simulink model "control_core"  (R2022b)
settings: Solver=FixedStepAuto  StartTime=0.0  StopTime=60  FixedStep=.01  RelTol=1e-3
undefined symbols (not defined in the file): airframe, CdProp, Cdx, Cdy, Cdz, Ct, Earth, g, Ixx, Iyy, Izz, Jr, larm, mass, WGS84
libraries: slpidlib x6, aerolibutil x3, vrlib x3, sharedtransform x2, shared6dof x2, simulink_extras x2, simulink x2, aerolibfltsims x1, aerolibtransform2 x1
(part 1 of 2)
settings Model: Creator=aaron  LastModifiedBy=aaron

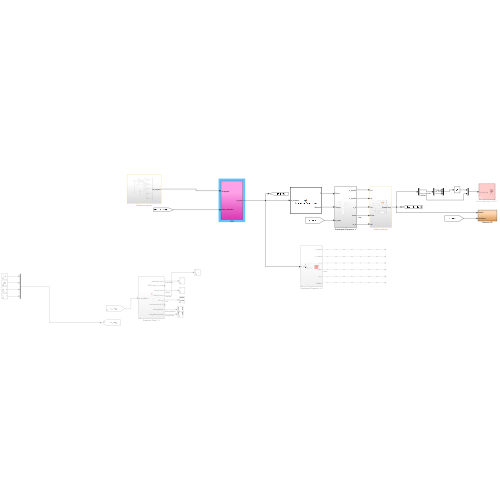
[thumbnail: Simulink's stored preview of the top-level diagram]
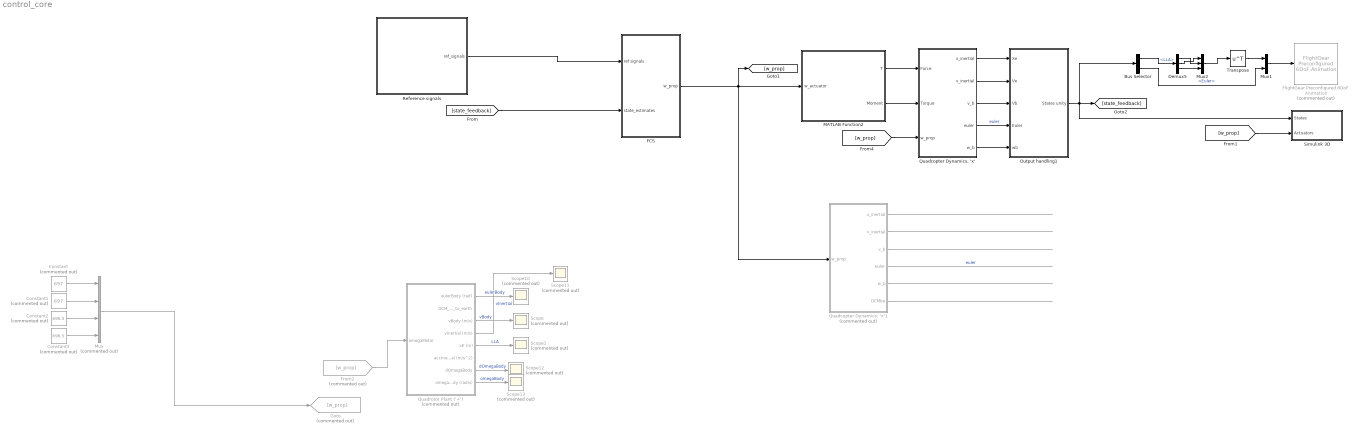
== system control_core ==
  Bus Selector : BusSelector  OutputSignals=LLA,Euler
  Constant : Constant  Commented=on  Value=697
  Constant1 : Constant  Commented=on  Value=697
  Constant2 : Constant  Commented=on  Value=696.5
  Constant3 : Constant  Commented=on  Value=696.5
  Demux5 : Demux  Outputs=3
  FCS : Subsystem
  FlightGear Preconfigured 6DoF Animation : aerolibfltsims/FlightGear Preconfigured 6DoF Animation  Commented=on  xFlightGearVersion=v2019.1  DestinationIpAddress=127.0.0.1  DestinationPort=5502  SampleTime=.0001  packetVersion=24
  From2 : From  Commented=on  GotoTag=w_prop
  Goto : Goto  Commented=on  GotoTag=w_prop
  MATLAB Function2 : MATLAB Function  TreatAsAtomicUnit=on
  Mux : Mux  Commented=on
  Mux1 : Mux  Inputs=2
  Mux2 : Mux  Inputs=3
  Output handling1 : Subsystem
  "Quadcopter Dynamics, 'x'" : Subsystem
  "Quadcopter Dynamics, 'x'1" : Subsystem  Commented=on
  Quadrotor Plant ('+') : Subsystem  Commented=on
  Reference signals : Subsystem
  Scope{,1,10..13} (6 alike) : Scope  Commented=on
  Simulink 3D : Subsystem  VariantControl=VSS_VISUALIZATION==VisualizationMode.Simulink_3D
  Transpose : Math  Operator=transpose
  wires:
  Quadrotor Plant ('+')/3(vBody (m/s)) -> Scope/1  "vBody"
  Quadrotor Plant ('+')/5(xE (m)) -> Scope1/1  "LLA"
  Mux/1 -> Goto/1
  Quadrotor Plant ('+')/1(eulerBody (rad)) -> Scope10/1  "eulerBody"
  Quadrotor Plant ('+')/4(vInertial (m/s)) -> Scope11/1  "vInertial"
  Quadrotor Plant ('+')/7(dOmegaBody) -> Scope12/1  "dOmegaBody"
  Quadrotor Plant ('+')/8(omegaBody (rad/s)) -> Scope13/1  "omegaBody"
  From2/1 -> Quadrotor Plant ('+')/1(omegaMotor)
  Constant/1 -> Mux/1
  Constant1/1 -> Mux/2
  Constant2/1 -> Mux/3
  Constant3/1 -> Mux/4
  "Quadcopter Dynamics, 'x'1"/1(x_inertial) -> ?
  "Quadcopter Dynamics, 'x'1"/2(v_inertial) -> ?
  "Quadcopter Dynamics, 'x'1"/3(v_b) -> ?
  "Quadcopter Dynamics, 'x'1"/4(euler) -> ?  "euler"
  "Quadcopter Dynamics, 'x'1"/5(w_b) -> ?
  "Quadcopter Dynamics, 'x'1"/6(DCMbe) -> ?
  MATLAB Function2/1(T) -> "Quadcopter Dynamics, 'x'"/1(Force)
  MATLAB Function2/2(Moment) -> "Quadcopter Dynamics, 'x'"/2(Torque)
  [w_prop] -> "Quadcopter Dynamics, 'x'"/3(w_prop)
  "Quadcopter Dynamics, 'x'"/1(x_inertial) -> Output handling1/1(Xe)
  "Quadcopter Dynamics, 'x'"/2(v_inertial) -> Output handling1/2(Ve)
  "Quadcopter Dynamics, 'x'"/3(v_b) -> Output handling1/3(Vb)
  "Quadcopter Dynamics, 'x'"/4(euler) -> Output handling1/4(Euler)  "euler"
  "Quadcopter Dynamics, 'x'"/5(w_b) -> Output handling1/5(wb)
  Output handling1/1(States unity) -> [state_feedback], Simulink 3D/1(States), Bus Selector/1
  Mux1/1 -> FlightGear Preconfigured 6DoF Animation/1
  Transpose/1 -> Mux1/1
  Demux5/1 -> Mux2/2
  Demux5/2 -> Mux2/1
  Mux2/1 -> Transpose/1
  Demux5/3 -> Mux2/3
  Bus Selector/1 -> Demux5/1  "<LLA>"
  Bus Selector/2 -> Mux1/2  "<Euler>"
  [w_prop] -> Simulink 3D/2(Actuators)
  FCS/1(w_prop) -> "Quadcopter Dynamics, 'x'1"/1(w_prop), [w_prop], MATLAB Function2/1(w_actuator)
  Reference signals/1(ref_signals) -> FCS/1(ref signals)
  [state_feedback] -> FCS/2(state_estimates)

== system control_core/FCS ==
  ref signals : Inport
  state_estimates : Inport  Port=2
  FCS : Subsystem
  Motor Mixing : Subsystem
  w_prop : Outport
  wires:
  ref signals/1 -> FCS/1(ref signals)
  FCS/2(Torque command) -> Motor Mixing/2(Torque)
  Motor Mixing/1(motor_rpm) -> w_prop/1  "w_prop"
  FCS/1(Force command) -> Motor Mixing/1(Force)
  state_estimates/1 -> FCS/2(state_estimates)

== system control_core/Output handling1 ==
  Xe : Inport
  Ve : Inport  Port=2
  Vb : Inport  Port=3
  Euler : Inport  Port=4
  wb : Inport  Port=5
  Bus Creator : BusCreator  Inputs=7
  Position on Earth : Subsystem  Priority=1  TreatAsAtomicUnit=on
  Rotation Angles to Direction Cosine Matrix : sharedtransform/Rotation Angles to Direction Cosine Matrix  rotationOrder=ZYX  aMode=aMode
  Selector : Selector  InputPortWidth=3  IndexOptions=Index vector (dialog)  Indices=[3 2 1]  OutputSizes=1
  States unity : Outport
  wires:
  Selector/1 -> Rotation Angles to Direction Cosine Matrix/1
  Bus Creator/1 -> States unity/1
  Ve/1 -> Bus Creator/3  "V_inertial"
  Xe/1 -> Position on Earth/1(Xe), Bus Creator/1  "X_inertial_me"
  Vb/1 -> Bus Creator/4  "v_body"
  wb/1 -> Bus Creator/6  "w_body"
  Euler/1 -> Bus Creator/5, Selector/1  "Euler"
  Rotation Angles to Direction Cosine Matrix/1 -> Bus Creator/7  "DCMbe"
  Position on Earth/1(LLA) -> Bus Creator/2  "LLA"

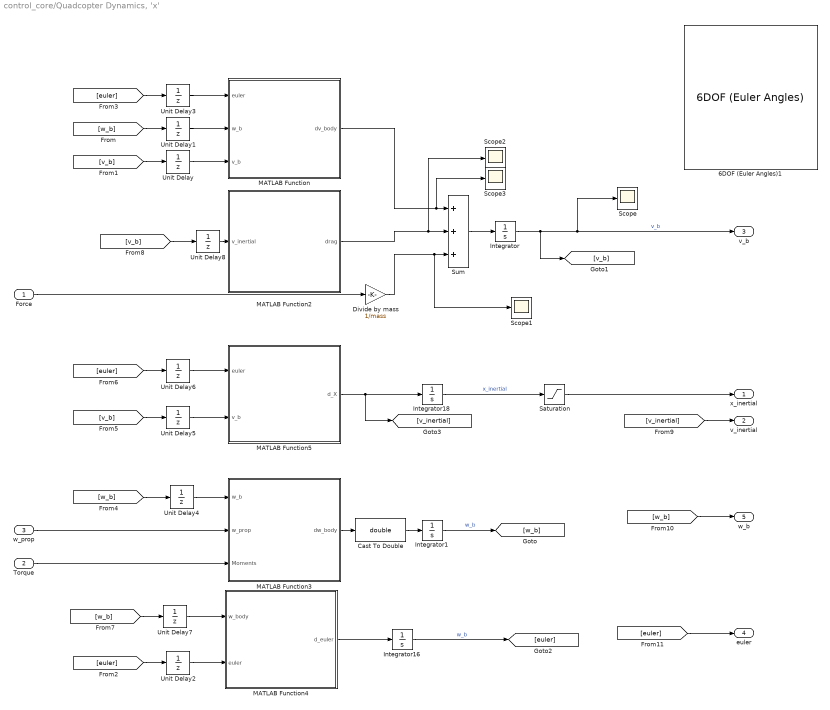
== system control_core/Quadcopter Dynamics, 'x' ==
  Force : Inport
  Torque : Inport  Port=2
  w_prop : Inport  Port=3
  6DOF (Euler Angles)1 : shared6dof/6DOF (Euler Angles)  units=Metric (MKS)  mtype=Fixed  rep=Euler Angles  xme_0=[0 0 0]  Vm_0=[0 0 0]  eul_0=[0 0 0]  pm_0=[0 0 0]  mass_0=1.0  mass_e=0.5  mass_f=2.0  inertia=eye(3)  inertia_e=eye(3)  inertia_f=2*eye(3)  k_quat=1.0  vre_flag=on  abi_flag=off  aMode=0  xme_statename=''  Vm_statename=''  eul_statename=''  quat_statename=''  pm_statename=''  mass_statename=''
  Cast To Double : DataTypeConversion  OutDataTypeStr=double  SaturateOnIntegerOverflow=off  RndMeth=Floor
  Divide by mass : Gain  Gain=1/mass
  Integrator : Integrator
  Integrator1 : Integrator
  Integrator16 : Integrator  InitialCondition=[0 0 0]  WrapState=on
  Integrator18 : Integrator  LimitOutput=on  UpperSaturationLimit=[inf inf 0]  LowerSaturationLimit=[-inf -inf -inf]
  MATLAB Function : MATLAB Function  TreatAsAtomicUnit=on
  MATLAB Function2 : MATLAB Function  TreatAsAtomicUnit=on
  MATLAB Function3 : MATLAB Function  TreatAsAtomicUnit=on
  MATLAB Function4 : MATLAB Function  TreatAsAtomicUnit=on
  MATLAB Function5 : MATLAB Function  TreatAsAtomicUnit=on
  Saturation : Saturate  UpperLimit=[inf inf 0]  LowerLimit=-inf
  Scope{,1..3} (4 alike) : Scope
  Sum : Sum  Inputs=+++
  Unit Delay{,1..8} (9 alike) : UnitDelay  SampleTime=-1  HasFrameUpgradeWarning=on
  x_inertial : Outport
  v_inertial : Outport  Port=2
  v_b : Outport  Port=3
  euler : Outport  Port=4
  w_b : Outport  Port=5
  wires:
  MATLAB Function/1(dv_body) -> Scope3/1, Sum/1
  MATLAB Function2/1(drag) -> Scope2/1, Sum/2
  Unit Delay/1 -> MATLAB Function/3(v_b)
  Force/1 -> Divide by mass/1
  MATLAB Function3/1(dw_body) -> Cast To Double/1
  Sum/1 -> Integrator/1
  Integrator1/1 -> [w_b]  "w_b"
  Unit Delay1/1 -> MATLAB Function/2(w_b)
  [w_b] -> Unit Delay1/1
  Integrator/1 -> Scope/1, v_b/1, [v_b]  "v_b"
  [v_b] -> Unit Delay/1
  MATLAB Function4/1(d_euler) -> Integrator16/1
  Integrator16/1 -> [euler]  "w_b"
  Unit Delay2/1 -> MATLAB Function4/2(euler)
  [euler] -> Unit Delay3/1
  Unit Delay3/1 -> MATLAB Function/1(euler)
  [euler] -> Unit Delay2/1
  w_prop/1 -> MATLAB Function3/2(w_prop)
  [w_b] -> Unit Delay4/1
  Unit Delay4/1 -> MATLAB Function3/1(w_b)
  [v_b] -> Unit Delay5/1
  Unit Delay5/1 -> MATLAB Function5/2(v_b)
  [euler] -> Unit Delay6/1
  Unit Delay6/1 -> MATLAB Function5/1(euler)
  [w_b] -> Unit Delay7/1
  Unit Delay7/1 -> MATLAB Function4/1(w_body)
  MATLAB Function5/1(d_X) -> Integrator18/1, [v_inertial]
  Unit Delay8/1 -> MATLAB Function2/1(v_inertial)
  [v_b] -> Unit Delay8/1
  [v_inertial] -> v_inertial/1
  Integrator18/1 -> Saturation/1  "x_inertial"
  Saturation/1 -> x_inertial/1
  [w_b] -> w_b/1
  [euler] -> euler/1
  Cast To Double/1 -> Integrator1/1
  Torque/1 -> MATLAB Function3/3(Moments)
  Divide by mass/1 -> Scope1/1, Sum/3

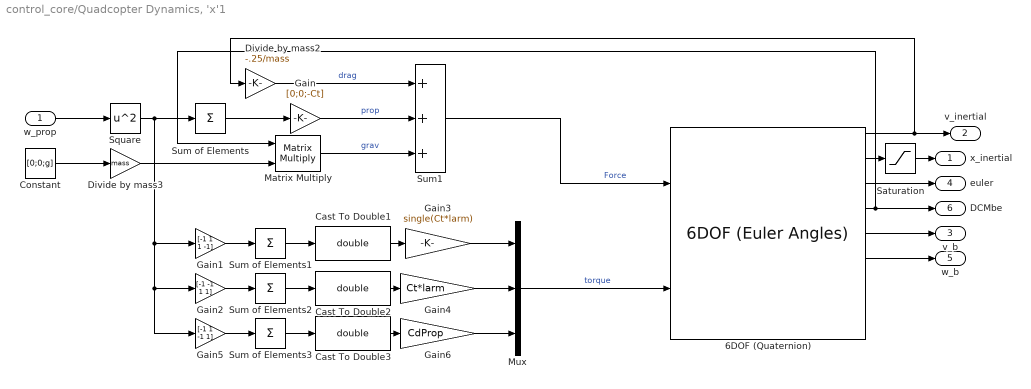
== system control_core/Quadcopter Dynamics, 'x'1 ==
  w_prop : Inport
  6DOF (Quaternion) : shared6dof/6DOF (Euler Angles)  units=Metric (MKS)  mtype=Fixed  rep=Euler Angles  xme_0=[0,0,0]  Vm_0=[0,0,0]  eul_0=[0,0,0]  pm_0=[0,0,0]  mass_0=mass  mass_e=0.5  mass_f=2.0  inertia=diag([Ixx Iyy Izz])  inertia_e=eye(3)  inertia_f=2*eye(3)  k_quat=Vehicle.SixDOF.quatGain  vre_flag=on  abi_flag=on  aMode=aMode  xme_statename=''  Vm_statename=''  eul_statename=''  quat_statename=''  pm_statename=''  mass_statename=''
  Cast To Double1 : DataTypeConversion  OutDataTypeStr=double  SaturateOnIntegerOverflow=off  RndMeth=Floor
  Cast To Double2 : DataTypeConversion  OutDataTypeStr=double  SaturateOnIntegerOverflow=off  RndMeth=Floor
  Cast To Double3 : DataTypeConversion  OutDataTypeStr=double  SaturateOnIntegerOverflow=off  RndMeth=Floor
  Constant : Constant  Value=[0;0;g]
  Divide by mass2 : Gain  Gain=-.25/mass
  Divide by mass3 : Gain  Gain=mass
  Gain : Gain  Gain=[0;0;-Ct]
  Gain1 : Gain  Gain=[-1 1 1 -1]
  Gain2 : Gain  Gain=[-1 -1 1 1]
  Gain3 : Gain  Gain=single(Ct*larm)
  Gain4 : Gain  Gain=Ct*larm
  Gain5 : Gain  Gain=[-1 1 -1 1]
  Gain6 : Gain  Gain=CdProp
  Matrix Multiply : Product  Multiplication=Matrix(*)
  Mux : Mux  Inputs=3
  Saturation : Saturate  UpperLimit=[inf inf 0]  LowerLimit=-inf
  Square : Math  Operator=square
  Sum of Elements{,1..3} (4 alike) : Sum  Inputs=+
  Sum1 : Sum  Inputs=+++
  x_inertial : Outport
  v_inertial : Outport  Port=2
  v_b : Outport  Port=3
  euler : Outport  Port=4
  w_b : Outport  Port=5
  DCMbe : Outport  Port=6
  wires:
  Sum1/1 -> 6DOF (Quaternion)/1  "Force"
  Constant/1 -> Divide by mass3/1
  6DOF (Quaternion)/1 -> v_inertial/1, Divide by mass2/1
  Divide by mass2/1 -> Sum1/1  "drag"
  w_prop/1 -> Square/1
  Square/1 -> Gain5/1, Gain2/1, Gain1/1, Sum of Elements/1
  Sum of Elements/1 -> Gain/1
  Gain/1 -> Sum1/2  "prop"
  Gain1/1 -> Sum of Elements1/1
  Gain2/1 -> Sum of Elements2/1
  Gain5/1 -> Sum of Elements3/1
  Gain3/1 -> Mux/1
  Gain4/1 -> Mux/2
  Gain6/1 -> Mux/3
  Mux/1 -> 6DOF (Quaternion)/2  "torque"
  6DOF (Quaternion)/5 -> v_b/1
  6DOF (Quaternion)/2 -> Saturation/1
  6DOF (Quaternion)/6 -> w_b/1
  6DOF (Quaternion)/3 -> euler/1
  6DOF (Quaternion)/4 -> Matrix Multiply/1, DCMbe/1
  Cast To Double1/1 -> Gain3/1
  Sum of Elements1/1 -> Cast To Double1/1
  Cast To Double2/1 -> Gain4/1
  Sum of Elements2/1 -> Cast To Double2/1
  Sum of Elements3/1 -> Cast To Double3/1
  Cast To Double3/1 -> Gain6/1
  Saturation/1 -> x_inertial/1
  Divide by mass3/1 -> Matrix Multiply/2
  Matrix Multiply/1 -> Sum1/3  "grav"

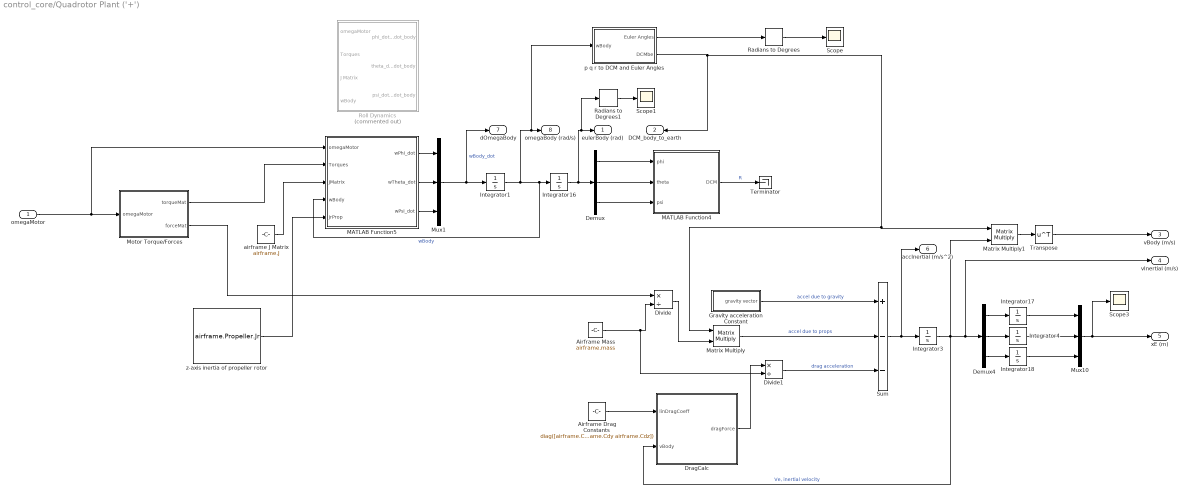
== system control_core/Quadrotor Plant ('+') ==
  omegaMotor : Inport
  Airframe Drag Constants : Constant  Value=diag([airframe.Cdx airframe.Cdy airframe.Cdz])
  Airframe Mass : Constant  Value=airframe.mass
  Demux : Demux  Outputs=3
  Demux4 : Demux  Outputs=3
  Divide : Product  Inputs=*/
  Divide1 : Product  Inputs=*/
  DragCalc : Subsystem
  Gravity acceleration Constant : Subsystem
  Integrator1 : Integrator  InitialCondition=[0 0 0]
  Integrator16 : Integrator  WrapState=on
  Integrator17 : Integrator
  Integrator18 : Integrator  LimitOutput=on  UpperSaturationLimit=0
  Integrator3 : Integrator
  Integrator4 : Integrator
  MATLAB Function4 : MATLAB Function  TreatAsAtomicUnit=on
  MATLAB Function5 : MATLAB Function  TreatAsAtomicUnit=on
  Matrix Multiply : Product  Multiplication=Matrix(*)
  Matrix Multiply1 : Product  Multiplication=Matrix(*)
  Motor Torque/Forces : Subsystem
  Mux1 : Mux  Inputs=3
  Mux10 : Mux  Inputs=3
  Radians to Degrees : simulink_extras/Transformations/Radians to Degrees
  Radians to Degrees1 : simulink_extras/Transformations/Radians to Degrees
  Roll Dynamics : Subsystem  Commented=on
  Scope : Scope
  Scope1 : Scope
  Scope3 : Scope
  Sum : Sum  Inputs=+--
  Terminator : Terminator
  Transpose : Math  Operator=transpose
  airframe J Matrix : Constant  Value=airframe.J
  p q r to DCM and Euler Angles : Subsystem
  z-axis inertia of propeller rotor : Constant  Value=airframe.Propeller.Jr
  eulerBody (rad) : Outport
  DCM_body_to_earth : Outport  Port=2
  vBody (m/s) : Outport  Port=3
  vInertial (m/s) : Outport  Port=4
  xE (m) : Outport  Port=5
  accInertial (m/s^2) : Outport  Port=6
  dOmegaBody : Outport  Port=7
  omegaBody (rad/s) : Outport  Port=8
  wires:
  Motor Torque/Forces/1(torqueMat) -> MATLAB Function5/2(Torques)
  omegaMotor/1 -> MATLAB Function5/1(omegaMotor), Motor Torque/Forces/1(omegaMotor)
  Integrator1/1 -> p q r to DCM and Euler Angles/1(wBody), omegaBody (rad/s)/1, MATLAB Function5/4(wBody), Integrator16/1  "wBody"
  Motor Torque/Forces/2(forceMat) -> Divide/1
  Airframe Mass/1 -> Divide1/2, Divide/2
  Divide/1 -> Matrix Multiply/2
  Matrix Multiply/1 -> Sum/2  "accel due to props"
  Gravity acceleration Constant/1(gravity vector) -> Sum/1  "accel due to gravity"
  DragCalc/1(dragForce) -> Divide1/1
  Sum/1 -> Integrator3/1, accInertial (m/s^2)/1
  Integrator3/1 -> Matrix Multiply1/2, vInertial (m/s)/1, Demux4/1, DragCalc/2(vBody)  "Ve, inertial velocity"
  Airframe Drag Constants/1 -> DragCalc/1(linDragCoeff)
  Matrix Multiply1/1 -> Transpose/1
  Mux10/1 -> Scope3/1, xE (m)/1
  Mux1/1 -> dOmegaBody/1, Integrator1/1  "wBody_dot"
  Demux/1 -> MATLAB Function4/1(phi)
  Demux/2 -> MATLAB Function4/2(theta)
  Demux/3 -> MATLAB Function4/3(psi)
  Integrator16/1 -> Demux/1, Radians to Degrees1/1, eulerBody (rad)/1
  Demux4/1 -> Integrator17/1
  Demux4/2 -> Integrator4/1
  Demux4/3 -> Integrator18/1
  Integrator4/1 -> Mux10/2
  Integrator17/1 -> Mux10/1
  p q r to DCM and Euler Angles/1(Euler Angles) -> Radians to Degrees/1
  airframe J Matrix/1 -> MATLAB Function5/3(JMatrix)
  MATLAB Function5/1(wPhi_dot) -> Mux1/1
  MATLAB Function5/2(wTheta_dot) -> Mux1/2
  MATLAB Function5/3(wPsi_dot) -> Mux1/3
  z-axis inertia of propeller rotor/1 -> MATLAB Function5/5(JrProp)
  Transpose/1 -> vBody (m/s)/1
  Radians to Degrees/1 -> Scope/1
  p q r to DCM and Euler Angles/2(DCMbe) -> Matrix Multiply/1, Matrix Multiply1/1, DCM_body_to_earth/1
  MATLAB Function4/1(DCM) -> Terminator/1  "R"
  Radians to Degrees1/1 -> Scope1/1
  Integrator18/1 -> Mux10/3
  Divide1/1 -> Sum/3  "drag acceleration"

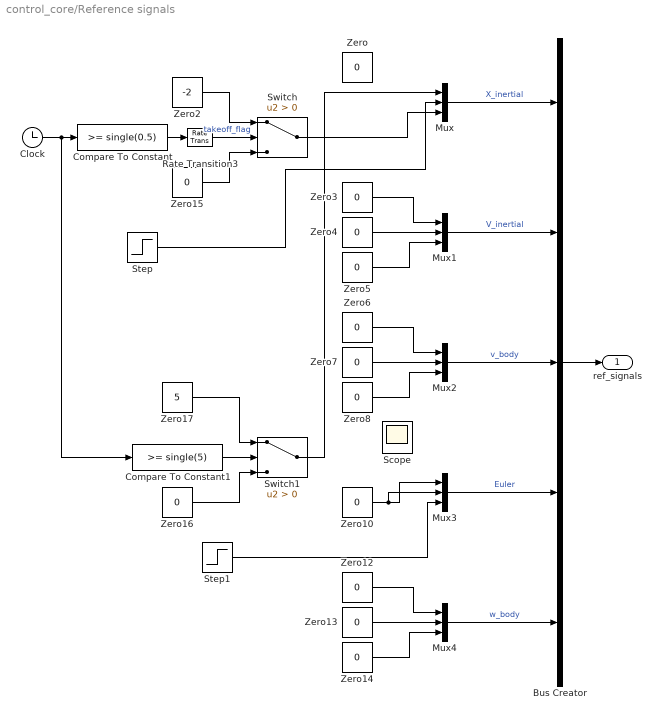
== system control_core/Reference signals ==
  Bus Creator : BusCreator  Inputs=5
  Clock : Clock
  Compare To Constant : simulink/Logic and Bit Operations/Compare To Constant  relop=>=  const=single(0.5)  OutDataTypeStr=boolean
  Compare To Constant1 : simulink/Logic and Bit Operations/Compare To Constant  relop=>=  const=single(5)  OutDataTypeStr=boolean
  Mux{,1..4} (5 alike) : Mux  Inputs=3
  Rate Transition3 : RateTransition  OutPortSampleTime=.01
  Scope : Scope
  Step : Step  Time=10  After=5  SampleTime=0
  Step1 : Step  Time=10  After=pi/24  SampleTime=0
  Switch : Switch  Criteria=u2 > Threshold  SaturateOnIntegerOverflow=off  InputSameDT=off
  Switch1 : Switch  Criteria=u2 > Threshold  SaturateOnIntegerOverflow=off  InputSameDT=off
  Zero{,3..8,10,12..16} (13 alike) : Constant  Value=0  OutDataTypeStr=Inherit: Inherit via back propagation
  Zero17 : Constant  Value=5  OutDataTypeStr=Inherit: Inherit via back propagation
  Zero2 : Constant  Value=-2  OutDataTypeStr=Inherit: Inherit via back propagation
  ref_signals : Outport
  wires:
  Mux3/1 -> Bus Creator/4  "Euler"
  Mux4/1 -> Bus Creator/5  "w_body"
  Mux2/1 -> Bus Creator/3  "v_body"
  Mux/1 -> Bus Creator/1  "X_inertial"
  Mux1/1 -> Bus Creator/2  "V_inertial"
  Bus Creator/1 -> ref_signals/1
  Zero5/1 -> Mux1/3
  Zero3/1 -> Mux1/1
  Zero4/1 -> Mux1/2
  Zero7/1 -> Mux2/2
  Zero8/1 -> Mux2/3
  Zero6/1 -> Mux2/1
  Zero13/1 -> Mux4/2
  Zero14/1 -> Mux4/3
  Zero12/1 -> Mux4/1
  Zero15/1 -> Switch/3
  Zero2/1 -> Switch/1
  Clock/1 -> Compare To Constant1/1, Compare To Constant/1
  Compare To Constant/1 -> Rate Transition3/1
  Rate Transition3/1 -> Switch/2  "takeoff_flag"
  Compare To Constant1/1 -> Switch1/2
  Zero16/1 -> Switch1/3
  Zero17/1 -> Switch1/1
  Switch/1 -> Mux/3
  Step/1 -> Mux/2
  Step1/1 -> Mux3/3
  Zero10/1 -> Mux3/2, Mux3/1
  Switch1/1 -> Mux/1

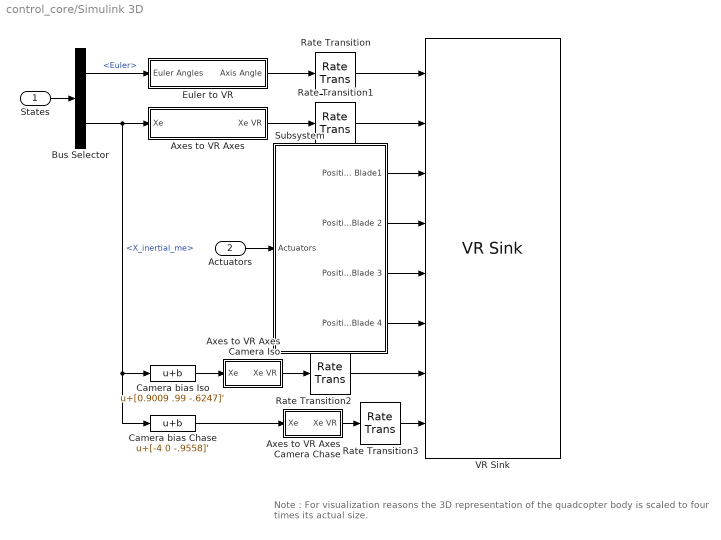
== system control_core/Simulink 3D ==
  note: Note : For visualization reasons the 3D representation of the quadcopter body is scaled to four times its actual size.
  States : Inport
  Actuators : Inport  Port=2
  Axes to VR Axes : Subsystem
  Axes to VR Axes Camera Chase : Subsystem
  Axes to VR Axes Camera Iso : Subsystem
  Bus Selector : BusSelector  OutputSignals=Euler,X_inertial_me
  Camera bias Chase : Bias  Bias=[-4 0 -.9558]'  SaturateOnIntegerOverflow=off
  Camera bias Iso : Bias  Bias=[0.9009 .99 -.6247]'  SaturateOnIntegerOverflow=off
  Euler to VR : Subsystem
  Rate Transition{,1..3} (4 alike) : RateTransition
  Subsystem : Subsystem
  VR Sink : vrlib/VR Sink  InstantiateOnLoad=on  SampleTime=10*.01  ViewEnable=on  RemoteChange=off  RemoteView=off  FieldsWritten=QuadBody.rotation.4.1.1.double#QuadBody.translation.3.1.1.double#Blade1.rotation.4.1.1.double#Blade2.rotation.4.1.1.double#Blade3.rotation.4.1.1.double#Blade4.rotation.4.1.1.double#IsoNoRotation.position.3.1.1.double#OnQuadNoRotation.position.3.1.1.double  WorldFileName=asbQuadcopterWorld.wrl  AutoView=on  VideoDimensions=[]  AllowVariableSize=off
  wires:
  Euler to VR/1(Axis Angle) -> Rate Transition/1
  Axes to VR Axes/1(Xe VR) -> Rate Transition1/1
  Bus Selector/1 -> Euler to VR/1(Euler Angles)  "<Euler>"
  Bus Selector/2 -> Axes to VR Axes/1(Xe), Camera bias Chase/1, Camera bias Iso/1  "<X_inertial_me>"
  States/1 -> Bus Selector/1
  Actuators/1 -> Subsystem/1(Actuators)
  Axes to VR Axes Camera Iso/1(Xe VR) -> Rate Transition2/1
  Camera bias Iso/1 -> Axes to VR Axes Camera Iso/1(Xe)
  Rate Transition/1 -> VR Sink/1
  Rate Transition1/1 -> VR Sink/2
  Subsystem/1(Position Blade1) -> VR Sink/3
  Subsystem/2(Position Blade 2) -> VR Sink/4
  Subsystem/3(Position Blade 3) -> VR Sink/5
  Subsystem/4(Position Blade 4) -> VR Sink/6
  Rate Transition2/1 -> VR Sink/7
  Axes to VR Axes Camera Chase/1(Xe VR) -> Rate Transition3/1
  Rate Transition3/1 -> VR Sink/8
  Camera bias Chase/1 -> Axes to VR Axes Camera Chase/1(Xe)

== system control_core/FCS/FCS ==
  ref signals : Inport
  state_estimates : Inport  Port=2
  inner_loop : Subsystem
  outer_loop : Subsystem
  Force command : Outport
  Torque command : Outport  Port=2
  wires:
  state_estimates/1 -> outer_loop/2(state_estimates), [state_estimates]
  ref signals/1 -> [ref_signals], outer_loop/1(ref signals)
  outer_loop/1(attitude_sp) -> inner_loop/1(attitude_sp)
  [state_estimates] -> inner_loop/2(state_estimates)
  inner_loop/1(torque) -> Torque command/1
  outer_loop/2(Thrust_cmd) -> [thrust_cmd]
  [thrust_cmd] -> Force command/1
  [ref_signals] -> inner_loop/3(ref_signals)

== system control_core/FCS/Motor Mixing ==
  Force : Inport
  Torque : Inport  Port=2
  Cast To Single : DataTypeConversion  OutDataTypeStr=single  SaturateOnIntegerOverflow=off  RndMeth=Floor
  MATLAB Function : MATLAB Function  TreatAsAtomicUnit=on
  Matrix Multiply : Product  Multiplication=Matrix(*)
  Mux : Mux  Inputs=2
  Saturation : Saturate  UpperLimit=2000  LowerLimit=0
  Scope : Scope
  SignedSqrt1 : Sqrt  Operator=signedSqrt  IntermediateResultsDataTypeStr=single
  motor_rpm : Outport
  wires:
  Torque/1 -> Mux/2  "torque"
  Force/1 -> Mux/1
  Saturation/1 -> motor_rpm/1
  SignedSqrt1/1 -> Saturation/1
  Matrix Multiply/1 -> SignedSqrt1/1
  MATLAB Function/1(controlMatInv) -> Matrix Multiply/1  "invcontrolMat"
  Cast To Single/1 -> Matrix Multiply/2
  Mux/1 -> Scope/1, Cast To Single/1

== system control_core/Output handling1/Position on Earth ==
  Xe : Inport  Unit=m
  Flat Earth to LLA : aerolibtransform2/Flat Earth to LLA  units=Metric (MKS)  ptype=Earth (WGS84)  F=1/298.257223563  R=6378137  refPosPort=off  LL0=[-122.389977, 37.615223]  psi=0
  Mux : Mux  Inputs=2
  href : Constant  Value=-4
  LLA : Outport  VectorParamsAs1DForOutWhenUnconnected=off
  wires:
  Mux/1 -> LLA/1
  Xe/1 -> Flat Earth to LLA/1
  Flat Earth to LLA/1 -> Mux/1
  Flat Earth to LLA/2 -> Mux/2
  href/1 -> Flat Earth to LLA/2

== system control_core/Quadrotor Plant ('+')/DragCalc ==
  linDragCoeff : Inport
  vBody : Inport  Port=2
  Matrix Multiply : Product  Multiplication=Matrix(*)
  dragForce : Outport
  wires:
  linDragCoeff/1 -> Matrix Multiply/1
  vBody/1 -> Matrix Multiply/2
  Matrix Multiply/1 -> dragForce/1

== system control_core/Quadrotor Plant ('+')/Gravity acceleration Constant ==
  Constant : Constant  Value=[0; 0; g]
  gravity vector : Outport
  wires:
  Constant/1 -> gravity vector/1

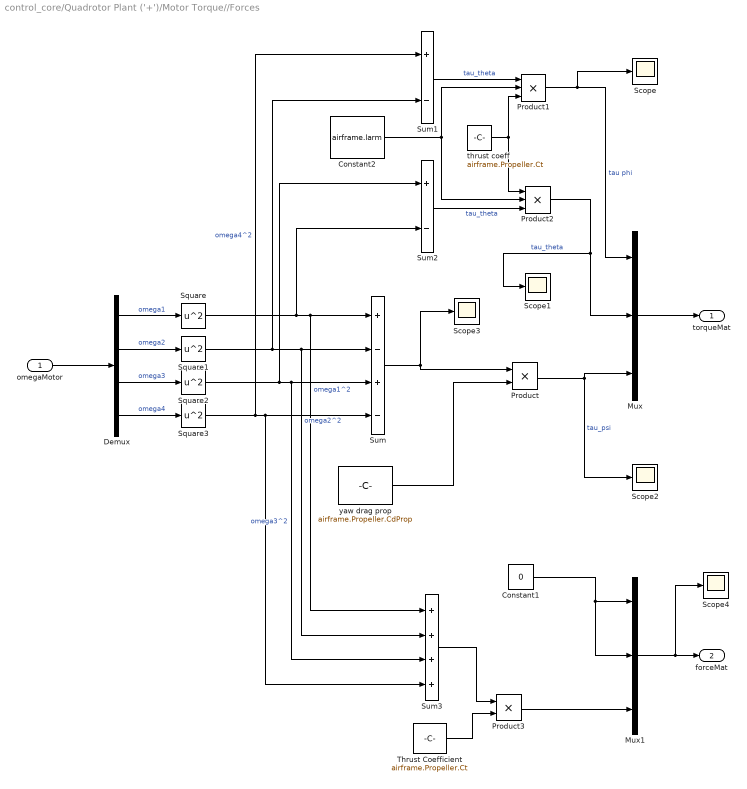
== system control_core/Quadrotor Plant ('+')/Motor Torque//Forces ==
  omegaMotor : Inport
  Constant1 : Constant  Value=0
  Constant2 : Constant  Value=airframe.larm
  Demux : Demux
  Mux : Mux  Inputs=3
  Mux1 : Mux  Inputs=3
  Product : Product
  Product1 : Product  Inputs=3
  Product2 : Product  Inputs=3
  Product3 : Product
  Scope{,1..4} (5 alike) : Scope
  Square{,1..3} (4 alike) : Math  Operator=square
  Sum : Sum  Inputs=+-+-
  Sum1 : Sum  Inputs=+-
  Sum2 : Sum  Inputs=+-
  Sum3 : Sum  Inputs=++++
  Thrust Coefficient : Constant  Value=airframe.Propeller.Ct
  thrust coeff : Constant  Value=airframe.Propeller.Ct
  yaw drag prop : Constant  Value=airframe.Propeller.CdProp
  torqueMat : Outport
  forceMat : Outport  Port=2
  wires:
  omegaMotor/1 -> Demux/1
  Demux/1 -> Square/1  "omega1"
  Demux/2 -> Square1/1  "omega2"
  Demux/3 -> Square2/1  "omega3"
  Demux/4 -> Square3/1  "omega4"
  Square2/1 -> Sum2/1, Sum3/3, Sum/3  "omega3^2"
  Square1/1 -> Sum1/2, Sum3/2, Sum/2  "omega2^2"
  Square/1 -> Sum2/2, Sum3/1, Sum/1  "omega1^2"
  Square3/1 -> Sum1/1, Sum3/4, Sum/4  "omega4^2"
  Sum/1 -> Scope3/1, Product/1
  Product/1 -> Mux/3, Scope2/1  "tau_psi"
  yaw drag prop/1 -> Product/2
  Product2/1 -> Mux/2, Scope1/1  "tau_theta"
  Product1/1 -> Scope/1, Mux/1  "tau phi"
  Constant2/1 -> Product2/2, Product1/2
  Sum1/1 -> Product1/1  "tau_theta"
  Mux/1 -> torqueMat/1
  Sum3/1 -> Product3/1
  Thrust Coefficient/1 -> Product3/2
  Mux1/1 -> Scope4/1, forceMat/1
  Product3/1 -> Mux1/3
  Constant1/1 -> Mux1/2, Mux1/1
  Sum2/1 -> Product2/3  "tau_theta"
  thrust coeff/1 -> Product1/3, Product2/1

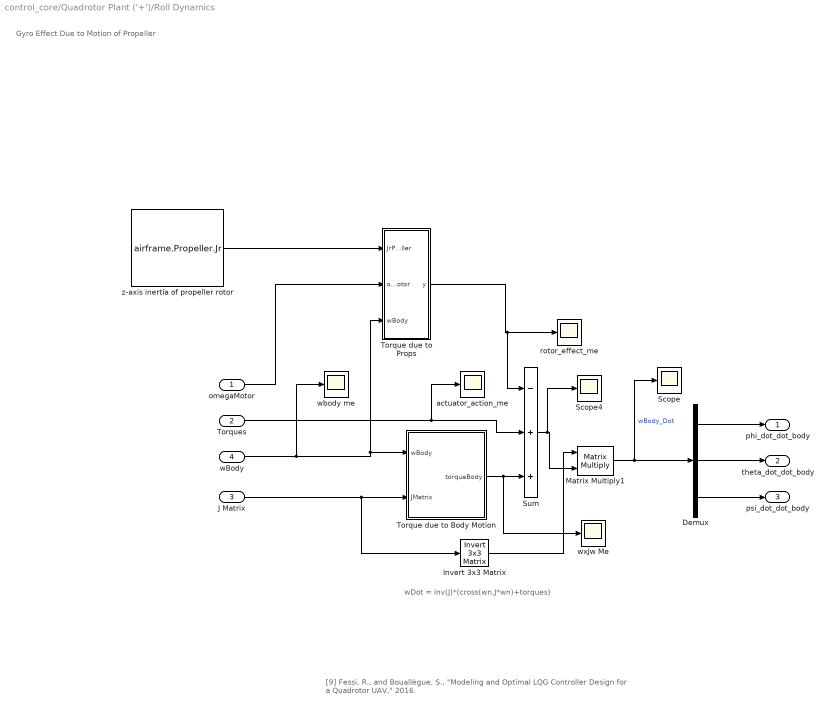
== system control_core/Quadrotor Plant ('+')/Roll Dynamics ==
  note: Gyro Effect Due to Motion of Propeller
  note: [9] Fessi, R., and Bouallègue, S., "Modeling and Optimal LQG Controller Design for a Quadrotor UAV," 2016.
  note: wDot = inv(J)*(cross(wn,J*wn)+torques)
  omegaMotor : Inport
  Torques : Inport  Port=2
  J Matrix : Inport  Port=3
  wBody : Inport  Port=4
  Demux : Demux  Outputs=3
  Invert 3x3 Matrix : aerolibutil/Invert  3x3 Matrix
  Matrix Multiply1 : Product  Multiplication=Matrix(*)
  Scope : Scope
  Scope4 : Scope
  Sum : Sum  Inputs=-++
  Torque due to Body Motion : Subsystem
  Torque due to Props : Subsystem
  actuator_action_me : Scope
  rotor_effect_me : Scope
  wbody me : Scope
  wxJw Me : Scope
  z-axis inertia of propeller rotor : Constant  Value=airframe.Propeller.Jr
  phi_dot_dot_body : Outport
  theta_dot_dot_body : Outport  Port=2
  psi_dot_dot_body : Outport  Port=3
  wires:
  wBody/1 -> wbody me/1, Torque due to Props/3(wBody), Torque due to Body Motion/1(wBody)
  J Matrix/1 -> Invert 3x3 Matrix/1, Torque due to Body Motion/2(JMatrix)
  Invert 3x3 Matrix/1 -> Matrix Multiply1/1
  Sum/1 -> Scope4/1, Matrix Multiply1/2
  Matrix Multiply1/1 -> Scope/1, Demux/1  "wBody_Dot"
  Demux/1 -> phi_dot_dot_body/1
  Demux/2 -> theta_dot_dot_body/1
  Demux/3 -> psi_dot_dot_body/1
  Torques/1 -> actuator_action_me/1, Sum/2
  z-axis inertia of propeller rotor/1 -> Torque due to Props/1(JrPropeller)
  omegaMotor/1 -> Torque due to Props/2(omegaMotor)
  Torque due to Props/1(y) -> Sum/1, rotor_effect_me/1
  Torque due to Body Motion/1(torqueBody) -> wxJw Me/1, Sum/3

== system control_core/Quadrotor Plant ('+')/p q r to DCM and Euler Angles ==
  wBody : Inport
  Integrator : Integrator  WrapState=on
  MATLAB Function : MATLAB Function  TreatAsAtomicUnit=on
  MATLAB Function1 : MATLAB Function  Commented=on  TreatAsAtomicUnit=on
  Rotation Angles to Direction Cosine Matrix : sharedtransform/Rotation Angles to Direction Cosine Matrix  rotationOrder=ZYX  aMode=aMode
  Scope : Scope
  Scope1 : Scope
  Selector : Selector  InputPortWidth=3  IndexOptions=Index vector (dialog)  Indices=[3 2 1]  OutputSizes=1
  Euler Angles : Outport
  DCMbe : Outport  Port=2
  wires:
  wBody/1 -> MATLAB Function/1(wBody)
  MATLAB Function/1(eulerAngleRates) -> Scope1/1, Integrator/1
  Selector/1 -> Rotation Angles to Direction Cosine Matrix/1
  Integrator/1 -> Selector/1, Scope/1, Euler Angles/1, MATLAB Function/2(eulerAngles)
  Rotation Angles to Direction Cosine Matrix/1 -> DCMbe/1

== system control_core/Simulink 3D/Axes to VR Axes ==
  Xe : Inport
  Constant : Constant  Value=50
  Constant1 : Constant  Value=.0460
  Constant2 : Constant  Value=95
  Demux : Demux  Outputs=3
      settings: DisplayOption=none
  Mux : Mux  Inputs=3
  Sum : Sum  Inputs=|++
  Sum1 : Sum  Inputs=|++
  Sum2 : Sum  Inputs=|++
  rad-->deg1 : Gain  Gain=-1  SaturateOnIntegerOverflow=on  OutDataTypeStr=Inherit: Same as input  ParamDataTypeStr=Inherit: Same as input
  Xe VR : Outport  VectorParamsAs1DForOutWhenUnconnected=off
  wires:
  Xe/1 -> Demux/1
  Demux/3 -> rad-->deg1/1
  Mux/1 -> Xe VR/1
  Demux/1 -> Sum/1
  Demux/2 -> Sum1/1
  rad-->deg1/1 -> Sum2/1
  Constant/1 -> Sum/2
  Sum/1 -> Mux/1
  Constant2/1 -> Sum1/2
  Constant1/1 -> Sum2/2
  Sum1/1 -> Mux/3
  Sum2/1 -> Mux/2

== system control_core/Simulink 3D/Axes to VR Axes Camera Chase ==
  Xe : Inport
  Demux : Demux  Outputs=3
      settings: DisplayOption=none
  Mux : Mux  Inputs=3
  rad-->deg1 : Gain  Gain=-1  SaturateOnIntegerOverflow=on  OutDataTypeStr=Inherit: Same as input  ParamDataTypeStr=Inherit: Same as input
  Xe VR : Outport  VectorParamsAs1DForOutWhenUnconnected=off
  wires:
  Xe/1 -> Demux/1
  Demux/1 -> Mux/1
  Demux/3 -> rad-->deg1/1
  Mux/1 -> Xe VR/1
  rad-->deg1/1 -> Mux/2
  Demux/2 -> Mux/3

== system control_core/Simulink 3D/Axes to VR Axes Camera Iso ==
  Xe : Inport
  Demux : Demux  Outputs=3
      settings: DisplayOption=none
  Mux : Mux  Inputs=3
  rad-->deg1 : Gain  Gain=-1  SaturateOnIntegerOverflow=on  OutDataTypeStr=Inherit: Same as input  ParamDataTypeStr=Inherit: Same as input
  Xe VR : Outport  VectorParamsAs1DForOutWhenUnconnected=off
  wires:
  Demux/2 -> Mux/3
  rad-->deg1/1 -> Mux/2
  Mux/1 -> Xe VR/1
  Demux/3 -> rad-->deg1/1
  Demux/1 -> Mux/1
  Xe/1 -> Demux/1

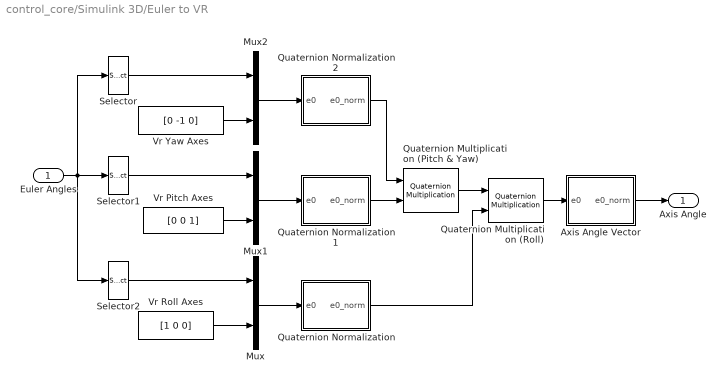
== system control_core/Simulink 3D/Euler to VR ==
  Euler Angles : Inport
  Axis Angle Vector : Subsystem
  Mux : Mux  Inputs=2
  Mux1 : Mux  Inputs=2
  Mux2 : Mux  Inputs=2
  Quaternion Multiplication (Pitch & Yaw) : aerolibutil/Quaternion Multiplication
  Quaternion Multiplication (Roll) : aerolibutil/Quaternion Multiplication
  Quaternion Normalization : Subsystem
  Quaternion Normalization1 : Subsystem
  Quaternion Normalization2 : Subsystem
  Selector : Selector  InputPortWidth=3  IndexOptions=Index vector (dialog)  Indices=[3]  OutputSizes=1
  Selector1 : Selector  InputPortWidth=3  IndexOptions=Index vector (dialog)  Indices=[2]  OutputSizes=1
  Selector2 : Selector  InputPortWidth=3  IndexOptions=Index vector (dialog)  Indices=[1]  OutputSizes=1
  Vr Pitch Axes : Constant  Value=[0 0 1]
  Vr Roll Axes : Constant  Value=[1 0 0]
  Vr Yaw Axes : Constant  Value=[0 -1 0]
  Axis Angle : Outport  VectorParamsAs1DForOutWhenUnconnected=off
  wires:
  Quaternion Multiplication (Roll)/1 -> Axis Angle Vector/1(e0)
  Axis Angle Vector/1(e0_norm) -> Axis Angle/1
  Quaternion Normalization/1(e0_norm) -> Quaternion Multiplication (Roll)/2
  Quaternion Normalization2/1(e0_norm) -> Quaternion Multiplication (Pitch & Yaw)/1
  Quaternion Normalization1/1(e0_norm) -> Quaternion Multiplication (Pitch & Yaw)/2
  Mux2/1 -> Quaternion Normalization2/1(e0)
  Mux1/1 -> Quaternion Normalization1/1(e0)
  Mux/1 -> Quaternion Normalization/1(e0)
  Selector/1 -> Mux2/1
  Vr Yaw Axes/1 -> Mux2/2
  Selector1/1 -> Mux1/1
  Vr Pitch Axes/1 -> Mux1/2
  Selector2/1 -> Mux/1
  Vr Roll Axes/1 -> Mux/2
  Euler Angles/1 -> Selector2/1, Selector1/1, Selector/1
  Quaternion Multiplication (Pitch & Yaw)/1 -> Quaternion Multiplication (Roll)/1

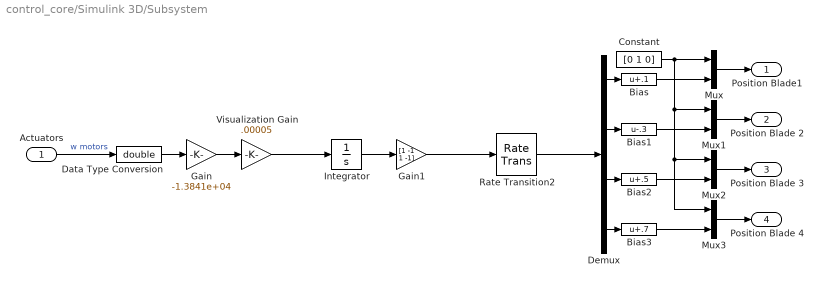
== system control_core/Simulink 3D/Subsystem ==
  Actuators : Inport
  Bias : Bias  Bias=.1  SaturateOnIntegerOverflow=off
  Bias1 : Bias  Bias=-.3  SaturateOnIntegerOverflow=off
  Bias2 : Bias  Bias=.5  SaturateOnIntegerOverflow=off
  Bias3 : Bias  Bias=.7  SaturateOnIntegerOverflow=off
  Constant : Constant  Value=[0 1 0]
  Data Type Conversion : DataTypeConversion  OutDataTypeStr=double  SaturateOnIntegerOverflow=off  RndMeth=Floor
  Demux : Demux
  Gain : Gain  Gain=-1.3841e+04
  Gain1 : Gain  Gain=[1 -1 1 -1]
  Integrator : Integrator  InitialCondition="[.1  .2 -.3 -.4]"  WrapState=on  WrappedStateUpperValue=2*pi  WrappedStateLowerValue=-2*pi
  Mux{,1..3} (4 alike) : Mux  Inputs=2
  Rate Transition2 : RateTransition
  Visualization Gain : Gain  Gain=.00005
  Position Blade1 : Outport  VectorParamsAs1DForOutWhenUnconnected=off
  Position Blade 2 : Outport  Port=2  VectorParamsAs1DForOutWhenUnconnected=off
  Position Blade 3 : Outport  Port=3  VectorParamsAs1DForOutWhenUnconnected=off
  Position Blade 4 : Outport  Port=4  VectorParamsAs1DForOutWhenUnconnected=off
  wires:
  Bias3/1 -> Mux3/2
  Mux3/1 -> Position Blade 4/1
  Bias1/1 -> Mux1/2
  Bias2/1 -> Mux2/2
  Demux/2 -> Bias1/1
  Visualization Gain/1 -> Integrator/1
  Constant/1 -> Mux3/1, Mux2/1, Mux1/1, Mux/1
  Mux1/1 -> Position Blade 2/1
  Mux2/1 -> Position Blade 3/1
  Data Type Conversion/1 -> Gain/1
  Mux/1 -> Position Blade1/1
  Gain/1 -> Visualization Gain/1
  Demux/3 -> Bias2/1
  Bias/1 -> Mux/2
  Actuators/1 -> Data Type Conversion/1  "w motors"
  Demux/4 -> Bias3/1
  Rate Transition2/1 -> Demux/1
  Demux/1 -> Bias/1
  Integrator/1 -> Gain1/1
  Gain1/1 -> Rate Transition2/1

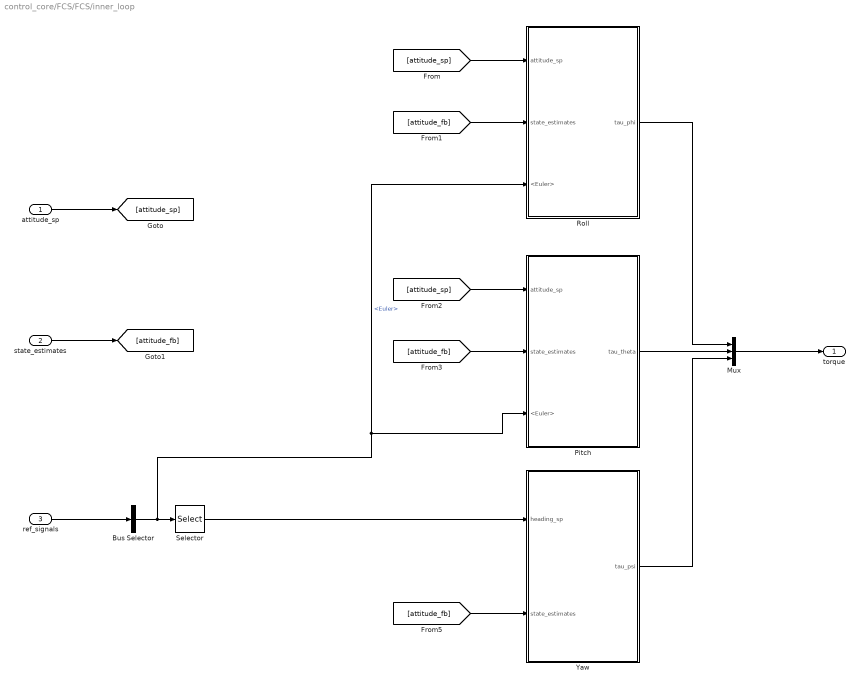
== system control_core/FCS/FCS/inner_loop ==
  attitude_sp : Inport
  state_estimates : Inport  Port=2
  ref_signals : Inport  Port=3
  Bus Selector : BusSelector  OutputSignals=Euler
  Mux : Mux  Inputs=3
  Pitch : Subsystem
  Roll : Subsystem
  Selector : Selector  InputPortWidth=3  IndexOptions=Index vector (dialog)  Indices=[3]  OutputSizes=1
  Yaw : Subsystem
  torque : Outport
  wires:
  attitude_sp/1 -> [attitude_sp]
  state_estimates/1 -> [attitude_fb]
  [attitude_sp] -> Roll/1(attitude_sp)
  [attitude_fb] -> Roll/2(state_estimates)
  [attitude_sp] -> Pitch/1(attitude_sp)
  [attitude_fb] -> Pitch/2(state_estimates)
  Selector/1 -> Yaw/1(heading_sp)
  [attitude_fb] -> Yaw/2(state_estimates)
  Roll/1(tau_phi) -> Mux/1
  Mux/1 -> torque/1
  Pitch/1(tau_theta) -> Mux/2
  ref_signals/1 -> Bus Selector/1
  Bus Selector/1 -> Pitch/3(<Euler>), Roll/3(<Euler>), Selector/1  "<Euler>"
  Yaw/1(tau_psi) -> Mux/3

== system control_core/FCS/FCS/outer_loop ==
  ref signals : Inport
  state_estimates : Inport  Port=2
  Altitude : Subsystem
  position : Subsystem
  attitude_sp : Outport
  Thrust_cmd : Outport  Port=2
  wires:
  position/1(pitch_roll_sp) -> attitude_sp/1
  Altitude/1(Thrust_cmd) -> Thrust_cmd/1
  ref signals/1 -> [ref_signals]
  state_estimates/1 -> [state_estimate]
  [ref_signals] -> position/1(ref signals)
  [state_estimate] -> position/2(state_estimates)
  [ref_signals] -> Altitude/1(ref_signals)
  [state_estimate] -> Altitude/2(state_estimates)

== system control_core/Quadrotor Plant ('+')/Roll Dynamics/Torque due to Body Motion ==
  wBody : Inport
  JMatrix : Inport  Port=2
  Cross Product : vrlib/Utilities/Cross Product
  Matrix Multiply : Product  Multiplication=Matrix(*)
  Scope : Scope
  Scope1 : Scope
  Scope2 : Scope
  torqueBody : Outport
  wires:
  Matrix Multiply/1 -> Cross Product/2, Scope2/1
  wBody/1 -> Matrix Multiply/2, Scope/1, Cross Product/1
  JMatrix/1 -> Matrix Multiply/1
  Cross Product/1 -> Scope1/1, torqueBody/1

== system control_core/Quadrotor Plant ('+')/Roll Dynamics/Torque due to Props ==
  JrPropeller : Inport
  omegaMotor : Inport  Port=2
  wBody : Inport  Port=3
  Cross Product1 : vrlib/Utilities/Cross Product
  Demux : Demux  Outputs=3
  Demux1 : Demux
  Gain : Gain  Gain=-1
  Mux : Mux  Inputs=3
  Mux1 : Mux  Inputs=3
  Product : Product
  Sum1 : Sum  Inputs=+-+-
  Zero1 : Constant  Value=0  OutDataTypeStr=Inherit: Inherit via back propagation
  y : Outport
  wires:
  Demux1/1 -> Sum1/1  "omega1"
  Demux1/2 -> Sum1/2  "omega2"
  Zero1/1 -> Mux1/2, Mux1/1
  Demux1/4 -> Sum1/4  "omega4"
  Product/1 -> Cross Product1/2  "Jr*Omega_R"
  Sum1/1 -> Product/2  "Omega_r"
  Demux1/3 -> Sum1/3  "omega3"
  Mux1/1 -> Product/1
  JrPropeller/1 -> Mux1/3
  wBody/1 -> Cross Product1/1
  omegaMotor/1 -> Demux1/1
  Cross Product1/1 -> Demux/1
  Mux/1 -> y/1
  Demux/1 -> Mux/1
  Demux/2 -> Gain/1
  Gain/1 -> Mux/2
  Demux/3 -> Mux/3

== system control_core/Simulink 3D/Euler to VR/Axis Angle Vector ==
  e0 : Inport
  2 : Gain  Gain=2  SaturateOnIntegerOverflow=on  OutDataTypeStr=Inherit: Same as input  ParamDataTypeStr=Inherit: Same as input
  Constant : Constant  Value=1e-6
  Demux : Demux  Outputs=[1 3 ]
      settings: DisplayOption=none
  Mux : Mux  Inputs=2
  Product : Product  Inputs=*/  InputSameDT=on  SaturateOnIntegerOverflow=on  OutDataTypeStr=Inherit: Same as first input
  Switch : Switch  Criteria=u2 ~= 0  SaturateOnIntegerOverflow=off  InputSameDT=off
  Trigonometric Function : Trigonometry
  Trigonometric Function2 : Trigonometry  Operator=acos
  e0_norm : Outport  VectorParamsAs1DForOutWhenUnconnected=off
  wires:
  Demux/1 -> Trigonometric Function2/1
  Demux/2 -> Product/1
  Mux/1 -> e0_norm/1
  Product/1 -> Mux/1
  2/1 -> Mux/2
  Trigonometric Function/1 -> Switch/1, Switch/2
  Trigonometric Function2/1 -> Trigonometric Function/1, 2/1
  e0/1 -> Demux/1
  Constant/1 -> Switch/3
  Switch/1 -> Product/2

== system control_core/Simulink 3D/Euler to VR/Quaternion Normalization ==
  e0 : Inport
  1/2 : Gain  Gain=1/2  SaturateOnIntegerOverflow=on  OutDataTypeStr=Inherit: Same as input  ParamDataTypeStr=Inherit: Same as input
  Demux : Demux  Outputs=[1 3]
      settings: DisplayOption=none
  Mux : Mux  Inputs=2
  Product : Product  InputSameDT=on  SaturateOnIntegerOverflow=on  OutDataTypeStr=Inherit: Same as first input
  Trigonometric Function : Trigonometry
  Trigonometric Function1 : Trigonometry  Operator=cos
  e0_norm : Outport  VectorParamsAs1DForOutWhenUnconnected=off
  wires:
  Trigonometric Function1/1 -> Mux/1
  Demux/2 -> Product/2
  Demux/1 -> 1/2/1
  Mux/1 -> e0_norm/1
  Product/1 -> Mux/2
  Trigonometric Function/1 -> Product/1
  1/2/1 -> Trigonometric Function1/1, Trigonometric Function/1
  e0/1 -> Demux/1

== system control_core/Simulink 3D/Euler to VR/Quaternion Normalization1 ==
  e0 : Inport
  1/2 : Gain  Gain=1/2  SaturateOnIntegerOverflow=on  OutDataTypeStr=Inherit: Same as input  ParamDataTypeStr=Inherit: Same as input
  Demux : Demux  Outputs=[1 3]
      settings: DisplayOption=none
  Mux : Mux  Inputs=2
  Product : Product  InputSameDT=on  SaturateOnIntegerOverflow=on  OutDataTypeStr=Inherit: Same as first input
  Trigonometric Function : Trigonometry
  Trigonometric Function1 : Trigonometry  Operator=cos
  e0_norm : Outport  VectorParamsAs1DForOutWhenUnconnected=off
  wires:
  e0/1 -> Demux/1
  1/2/1 -> Trigonometric Function/1, Trigonometric Function1/1
  Trigonometric Function/1 -> Product/1
  Product/1 -> Mux/2
  Mux/1 -> e0_norm/1
  Demux/1 -> 1/2/1
  Demux/2 -> Product/2
  Trigonometric Function1/1 -> Mux/1

== system control_core/Simulink 3D/Euler to VR/Quaternion Normalization2 ==
  e0 : Inport
  1/2 : Gain  Gain=1/2  SaturateOnIntegerOverflow=on  OutDataTypeStr=Inherit: Same as input  ParamDataTypeStr=Inherit: Same as input
  Demux : Demux  Outputs=[1 3]
      settings: DisplayOption=none
  Mux : Mux  Inputs=2
  Product : Product  InputSameDT=on  SaturateOnIntegerOverflow=on  OutDataTypeStr=Inherit: Same as first input
  Trigonometric Function : Trigonometry
  Trigonometric Function1 : Trigonometry  Operator=cos
  e0_norm : Outport  VectorParamsAs1DForOutWhenUnconnected=off
  wires:
  Trigonometric Function1/1 -> Mux/1
  Demux/2 -> Product/2
  Demux/1 -> 1/2/1
  Mux/1 -> e0_norm/1
  Product/1 -> Mux/2
  Trigonometric Function/1 -> Product/1
  1/2/1 -> Trigonometric Function1/1, Trigonometric Function/1
  e0/1 -> Demux/1

== system control_core/FCS/FCS/inner_loop/Pitch ==
  attitude_sp : Inport
  state_estimates : Inport  Port=2
  <Euler> : Inport  Port=3
  Bus Selector : BusSelector  OutputSignals=Euler
  PID Controller : slpidlib/PID Controller  Controller=PID  Form=Parallel  TimeDomain=Discrete-time  UseExternalTs=off  SampleTime=-1  IntegratorMethod=Forward Euler  FilterMethod=Forward Euler  ControllerParametersSource=internal  P=0.000755029982834631  I=1.9551161154067e-05  UseKiTs=off  D=0.00509235542495727  N=1.03816762728299  UseFilter=on  TunerSelectOption=Transfer Function Based (PID Tuner App)  InitialConditionSource=internal  InitialConditionForIntegrator=0  InitialConditionForFilter=0  DifferentiatorICPrevScaledInput=0  ExternalReset=none  TrackingMode=off  Kt=1  LimitOutput=off  SatLimitsSource=internal  UpperSaturationLimit=inf  LowerSaturationLimit=-inf  LinearizeAsGain=on  AntiWindupMode=clamping  Kb=1  LimitIntegrator=off  UpperIntegratorSaturationLimit=inf  LowerIntegratorSaturationLimit=-inf  POutMin=[]  POutMax=[]  IOutMin=[]  IOutMax=[]  DOutMin=[]  DOutMax=[]  NOutMin=[]  NOutMax=[]  SumOutMin=[]  SumOutMax=[]  SaturationOutMin=[]  SaturationOutMax=[]  PParamMin=[]  PParamMax=[]  IParamMin=[]  IParamMax=[]  DParamMin=[]  DParamMax=[]  NParamMin=[]  NParamMax=[]  KbParamMin=[]  KbParamMax=[]  KtParamMin=[]  KtParamMax=[]  KbOutMin=[]  KbOutMax=[]  KtOutMin=[]  KtOutMax=[]  IntegratorOutMin=[]  IntegratorOutMax=[]  FilterOutMin=[]  FilterOutMax=[]  SumI1OutMin=[]  SumI1OutMax=[]  SumI2OutMin=[]  SumI2OutMax=[]  SumI3OutMin=[]  SumI3OutMax=[]  SumI4OutMin=[]  SumI4OutMax=[]  SumDOutMin=[]  SumDOutMax=[]  DifferentiatorOutMin=[]  DifferentiatorOutMax=[]  FilterDiffOutCoefMin=[]  FilterDiffOutCoefMax=[]  ReciprocalOutMin=[]  ReciprocalOutMax=[]  SumDenOutMin=[]  SumDenOutMax=[]  SumNumOutMin=[]  SumNumOutMax=[]  DivideOutMin=[]  DivideOutMax=[]  UdiffTsProdOutMin=[]  UdiffTsProdOutMax=[]  NTsProdOutMin=[]  NTsProdOutMax=[]  UintegralTsProdOutMin=[]  UintegralTsProdOutMax=[]  UngainTsProdOutMin=[]  UngainTsProdOutMax=[]  ClampingZeroOutDataTypeStr=Inherit: Inherit via back propagation  ClampingZeroOutMin=[]  ClampingZeroOutMax=[]  FilterDenConstantOutDataTypeStr=Inherit: Inherit via back propagation  FilterDenConstantOutMin=[]  FilterDenConstantOutMax=[]  PCopyOutDataTypeStr=Inherit: Inherit via back propagation  PCopyOutMin=[]  PCopyOutMax=[]  NCopyOutDataTypeStr=Inherit: Inherit via back propagation  NCopyOutMin=[]  NCopyOutMax=[]  IntegratorContinuousStateAttributes=''  IntegratorStateMustResolveToSignalObject=off  IntegratorRTWStateStorageClass=Auto  FilterContinuousStateAttributes=''  FilterStateMustResolveToSignalObject=off  FilterRTWStateStorageClass=Auto  ParallelPVariant=InternalParameters  IdealPVariant=Disabled  IVariant=InternalParameters  DVariant=InternalParameters  IntegratorVariant=Discrete  SatVariant=Disabled  AWVariant=Passthrough  PCopyVariant=Disabled  TRVariant=Disabled  FdbkBlocksVariant=Forward  IdealPFdbkVariant=Disabled  SatFdbkVariant=Disabled  DerivativeFilterVariant=ForwardEulerFilter  NVariant=InternalParameters  NCopyVariant=Disabled  FilterICVariant=InternalICsFilter  IntegratorICVariant=InternalICs  ExternalResetVariant=Disabled  TRSumVariant=Passthrough  SumFdbkVariant=Disabled  SumVariant=Sum_PID  TsampFilterVariant=InternalTs  TsampNgainVariant=Passthrough  TsampIntegralVariant=Passthrough  ExternalSaturationOutDataTypeStr=Inherit: Same as second input
  Selector : Selector  InputPortWidth=2  IndexOptions=Index vector (dialog)  Indices=[2]  OutputSizes=1
  Selector1 : Selector  InputPortWidth=3  IndexOptions=Index vector (dialog)  Indices=[2]  OutputSizes=1
  Selector2 : Selector  InputPortWidth=3  IndexOptions=Index vector (dialog)  Indices=[2]  OutputSizes=1
  Sum : Sum  Inputs=|+-
  tau_theta : Outport
  wires:
  attitude_sp/1 -> Selector/1
  Sum/1 -> PID Controller/1
  PID Controller/1 -> tau_theta/1
  Bus Selector/1 -> Selector1/1  "<Euler>"
  Selector1/1 -> Sum/2
  state_estimates/1 -> Bus Selector/1
  <Euler>/1 -> Selector2/1
  Selector/1 -> Sum/1

== system control_core/FCS/FCS/inner_loop/Roll ==
  attitude_sp : Inport
  state_estimates : Inport  Port=2
  <Euler> : Inport  Port=3
  Bus Selector : BusSelector  OutputSignals=Euler
  PID Controller : slpidlib/PID Controller  Controller=PID  Form=Parallel  TimeDomain=Discrete-time  UseExternalTs=off  SampleTime=-1  IntegratorMethod=Forward Euler  FilterMethod=Forward Euler  ControllerParametersSource=internal  P=0.00222776202264695  I=2.18485015437245e-05  UseKiTs=off  D=0.0134340999324703  N=1.24748629813611  UseFilter=on  TunerSelectOption=Transfer Function Based (PID Tuner App)  InitialConditionSource=internal  InitialConditionForIntegrator=0  InitialConditionForFilter=0  DifferentiatorICPrevScaledInput=0  ExternalReset=none  TrackingMode=off  Kt=1  LimitOutput=off  SatLimitsSource=internal  UpperSaturationLimit=inf  LowerSaturationLimit=-inf  LinearizeAsGain=on  AntiWindupMode=clamping  Kb=1  LimitIntegrator=off  UpperIntegratorSaturationLimit=inf  LowerIntegratorSaturationLimit=-inf  POutMin=[]  POutMax=[]  IOutMin=[]  IOutMax=[]  DOutMin=[]  DOutMax=[]  NOutMin=[]  NOutMax=[]  SumOutMin=[]  SumOutMax=[]  SaturationOutMin=[]  SaturationOutMax=[]  PParamMin=[]  PParamMax=[]  IParamMin=[]  IParamMax=[]  DParamMin=[]  DParamMax=[]  NParamMin=[]  NParamMax=[]  KbParamMin=[]  KbParamMax=[]  KtParamMin=[]  KtParamMax=[]  KbOutMin=[]  KbOutMax=[]  KtOutMin=[]  KtOutMax=[]  IntegratorOutMin=[]  IntegratorOutMax=[]  FilterOutMin=[]  FilterOutMax=[]  SumI1OutMin=[]  SumI1OutMax=[]  SumI2OutMin=[]  SumI2OutMax=[]  SumI3OutMin=[]  SumI3OutMax=[]  SumI4OutMin=[]  SumI4OutMax=[]  SumDOutMin=[]  SumDOutMax=[]  DifferentiatorOutMin=[]  DifferentiatorOutMax=[]  FilterDiffOutCoefMin=[]  FilterDiffOutCoefMax=[]  ReciprocalOutMin=[]  ReciprocalOutMax=[]  SumDenOutMin=[]  SumDenOutMax=[]  SumNumOutMin=[]  SumNumOutMax=[]  DivideOutMin=[]  DivideOutMax=[]  UdiffTsProdOutMin=[]  UdiffTsProdOutMax=[]  NTsProdOutMin=[]  NTsProdOutMax=[]  UintegralTsProdOutMin=[]  UintegralTsProdOutMax=[]  UngainTsProdOutMin=[]  UngainTsProdOutMax=[]  ClampingZeroOutDataTypeStr=Inherit: Inherit via back propagation  ClampingZeroOutMin=[]  ClampingZeroOutMax=[]  FilterDenConstantOutDataTypeStr=Inherit: Inherit via back propagation  FilterDenConstantOutMin=[]  FilterDenConstantOutMax=[]  PCopyOutDataTypeStr=Inherit: Inherit via back propagation  PCopyOutMin=[]  PCopyOutMax=[]  NCopyOutDataTypeStr=Inherit: Inherit via back propagation  NCopyOutMin=[]  NCopyOutMax=[]  IntegratorContinuousStateAttributes=''  IntegratorStateMustResolveToSignalObject=off  IntegratorRTWStateStorageClass=Auto  FilterContinuousStateAttributes=''  FilterStateMustResolveToSignalObject=off  FilterRTWStateStorageClass=Auto  ParallelPVariant=InternalParameters  IdealPVariant=Disabled  IVariant=InternalParameters  DVariant=InternalParameters  IntegratorVariant=Discrete  SatVariant=Disabled  AWVariant=Passthrough  PCopyVariant=Disabled  TRVariant=Disabled  FdbkBlocksVariant=Forward  IdealPFdbkVariant=Disabled  SatFdbkVariant=Disabled  DerivativeFilterVariant=ForwardEulerFilter  NVariant=InternalParameters  NCopyVariant=Disabled  FilterICVariant=InternalICsFilter  IntegratorICVariant=InternalICs  ExternalResetVariant=Disabled  TRSumVariant=Passthrough  SumFdbkVariant=Disabled  SumVariant=Sum_PID  TsampFilterVariant=InternalTs  TsampNgainVariant=Passthrough  TsampIntegralVariant=Passthrough  ExternalSaturationOutDataTypeStr=Inherit: Same as second input
  Scope : Scope
  Scope2 : Scope
  Selector : Selector  InputPortWidth=2  IndexOptions=Index vector (dialog)  Indices=[1]  OutputSizes=1
  Selector1 : Selector  InputPortWidth=3  IndexOptions=Index vector (dialog)  Indices=[1]  OutputSizes=1
  Selector2 : Selector  InputPortWidth=3  IndexOptions=Index vector (dialog)  Indices=[1]  OutputSizes=1
  Sum : Sum  Inputs=|+-
  tau_phi : Outport
  wires:
  attitude_sp/1 -> Selector/1
  Sum/1 -> PID Controller/1, Scope/1
  Selector1/1 -> Sum/2
  PID Controller/1 -> Scope2/1, tau_phi/1
  state_estimates/1 -> Bus Selector/1
  Bus Selector/1 -> Selector1/1  "<Euler>"
  <Euler>/1 -> Selector2/1
  Selector/1 -> Sum/1

== system control_core/FCS/FCS/inner_loop/Yaw ==
  heading_sp : Inport
  state_estimates : Inport  Port=2
  Bus Selector : BusSelector  OutputSignals=Euler
  PID Controller : slpidlib/PID Controller  Controller=PD  Form=Parallel  TimeDomain=Discrete-time  UseExternalTs=off  SampleTime=-1  IntegratorMethod=Forward Euler  FilterMethod=Forward Euler  ControllerParametersSource=internal  P=0.00308709400862221  I=0  UseKiTs=off  D=0.020762699011989  N=9.31948574377754  UseFilter=on  TunerSelectOption=Transfer Function Based (PID Tuner App)  InitialConditionSource=internal  InitialConditionForIntegrator=0  InitialConditionForFilter=0  DifferentiatorICPrevScaledInput=0  ExternalReset=none  TrackingMode=off  Kt=1  LimitOutput=off  SatLimitsSource=internal  UpperSaturationLimit=inf  LowerSaturationLimit=-inf  LinearizeAsGain=on  AntiWindupMode=clamping  Kb=1  LimitIntegrator=off  UpperIntegratorSaturationLimit=inf  LowerIntegratorSaturationLimit=-inf  POutMin=[]  POutMax=[]  IOutMin=[]  IOutMax=[]  DOutMin=[]  DOutMax=[]  NOutMin=[]  NOutMax=[]  SumOutMin=[]  SumOutMax=[]  SaturationOutMin=[]  SaturationOutMax=[]  PParamMin=[]  PParamMax=[]  IParamMin=[]  IParamMax=[]  DParamMin=[]  DParamMax=[]  NParamMin=[]  NParamMax=[]  KbParamMin=[]  KbParamMax=[]  KtParamMin=[]  KtParamMax=[]  KbOutMin=[]  KbOutMax=[]  KtOutMin=[]  KtOutMax=[]  IntegratorOutMin=[]  IntegratorOutMax=[]  FilterOutMin=[]  FilterOutMax=[]  SumI1OutMin=[]  SumI1OutMax=[]  SumI2OutMin=[]  SumI2OutMax=[]  SumI3OutMin=[]  SumI3OutMax=[]  SumI4OutMin=[]  SumI4OutMax=[]  SumDOutMin=[]  SumDOutMax=[]  DifferentiatorOutMin=[]  DifferentiatorOutMax=[]  FilterDiffOutCoefMin=[]  FilterDiffOutCoefMax=[]  ReciprocalOutMin=[]  ReciprocalOutMax=[]  SumDenOutMin=[]  SumDenOutMax=[]  SumNumOutMin=[]  SumNumOutMax=[]  DivideOutMin=[]  DivideOutMax=[]  UdiffTsProdOutMin=[]  UdiffTsProdOutMax=[]  NTsProdOutMin=[]  NTsProdOutMax=[]  UintegralTsProdOutMin=[]  UintegralTsProdOutMax=[]  UngainTsProdOutMin=[]  UngainTsProdOutMax=[]  ClampingZeroOutDataTypeStr=Inherit: Inherit via back propagation  ClampingZeroOutMin=[]  ClampingZeroOutMax=[]  FilterDenConstantOutDataTypeStr=Inherit: Inherit via back propagation  FilterDenConstantOutMin=[]  FilterDenConstantOutMax=[]  PCopyOutDataTypeStr=Inherit: Inherit via back propagation  PCopyOutMin=[]  PCopyOutMax=[]  NCopyOutDataTypeStr=Inherit: Inherit via back propagation  NCopyOutMin=[]  NCopyOutMax=[]  IntegratorContinuousStateAttributes=''  IntegratorStateMustResolveToSignalObject=off  IntegratorRTWStateStorageClass=Auto  FilterContinuousStateAttributes=''  FilterStateMustResolveToSignalObject=off  FilterRTWStateStorageClass=Auto  ParallelPVariant=InternalParameters  IdealPVariant=Disabled  IVariant=Disabled  DVariant=InternalParameters  IntegratorVariant=Disabled  SatVariant=Disabled  AWVariant=Disabled  PCopyVariant=Disabled  TRVariant=Disabled  FdbkBlocksVariant=Forward  IdealPFdbkVariant=Disabled  SatFdbkVariant=Disabled  DerivativeFilterVariant=ForwardEulerFilter  NVariant=InternalParameters  NCopyVariant=Disabled  FilterICVariant=InternalICsFilter  IntegratorICVariant=Disabled  ExternalResetVariant=Disabled  TRSumVariant=Passthrough  SumFdbkVariant=Disabled  SumVariant=Sum_PD  TsampFilterVariant=InternalTs  TsampNgainVariant=Passthrough  TsampIntegralVariant=Disabled_SignalSpec  ExternalSaturationOutDataTypeStr=Inherit: Same as second input
  Selector1 : Selector  InputPortWidth=3  IndexOptions=Index vector (dialog)  Indices=[3]  OutputSizes=1
  Sum : Sum  Inputs=|+-
  tau_psi : Outport
  wires:
  heading_sp/1 -> Sum/1  "heading_sp"
  PID Controller/1 -> tau_psi/1
  Bus Selector/1 -> Selector1/1  "<Euler>"
  Selector1/1 -> Sum/2
  state_estimates/1 -> Bus Selector/1
  Sum/1 -> PID Controller/1

== system control_core/FCS/FCS/outer_loop/Altitude ==
  ref_signals : Inport
  state_estimates : Inport  Port=2
  Altitude PID : Subsystem
  Bus Selector : BusSelector  OutputSignals=X_inertial
  Bus Selector1 : BusSelector  OutputSignals=X_inertial_me,DCMbe
  Matrix Multiply : Product  Multiplication=Matrix(*)
  Matrix Multiply1 : Product  Multiplication=Matrix(*)
  Selector1 : Selector  InputPortWidth=3  IndexOptions=Index vector (dialog)  Indices=[3]  OutputSizes=1
  Selector2 : Selector  InputPortWidth=3  IndexOptions=Index vector (dialog)  Indices=[3]  OutputSizes=1
  Thrust_cmd : Outport
  wires:
  ref_signals/1 -> Bus Selector/1
  Bus Selector/1 -> Matrix Multiply/2  "<X_inertial>"
  state_estimates/1 -> Bus Selector1/1
  Bus Selector1/2 -> [DCMbe]  "<DCMbe>"
  [DCMbe] -> Matrix Multiply1/1, Matrix Multiply/1
  Bus Selector1/1 -> Matrix Multiply1/2  "<X_inertial_me>"
  Matrix Multiply1/1 -> Selector2/1
  Matrix Multiply/1 -> Selector1/1
  Selector1/1 -> Altitude PID/1(altitude_setpoint)
  Selector2/1 -> Altitude PID/2(altitude_feedback)
  Altitude PID/1(Out1) -> Thrust_cmd/1
